simulink model "zlinearyzowany_dyskretny_model_dynamiczny"  (R2021a)
settings: Solver=VariableStepAuto  StartTime=0.0  StopTime=60  RelTol=1e-3
values from neighbouring files (symbols this model uses):
  a1 = 0.32    [Wartosci_w_zadaniu.m]    (also in zad_4.m)
  a2 = 0.45    [Wartosci_w_zadaniu.m]    (also in zad_4.m)
  a3 = -0.29    [Wartosci_w_zadaniu.m]    (also in zad_4.m)
  a4 = -0.1    [Wartosci_w_zadaniu.m]    (also in zad_4.m)
  K = 2    [Wartosci_w_zadaniu.m]    (also in zad_4.m)
  T = 1.5    [zad_4.m]
  T1 = 5    [Wartosci_w_zadaniu.m]    (also in zad_4.m)
  T2 = 8    [Wartosci_w_zadaniu.m]    (also in zad_4.m)
  u_0 = -0.85    [zad_5_i_6.m]
settings Model: Creator=ADMIN  LastModifiedBy=ADMIN

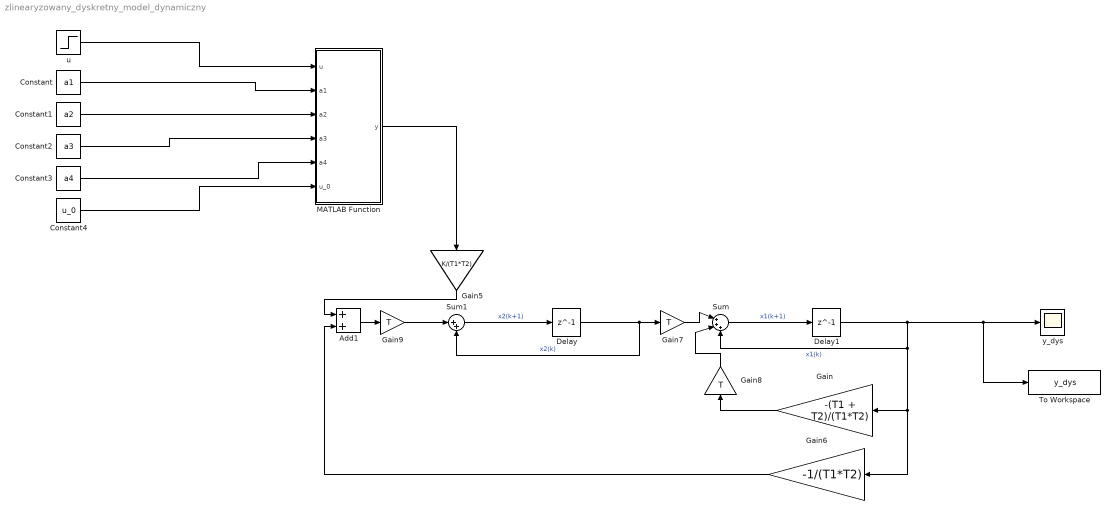
== system zlinearyzowany_dyskretny_model_dynamiczny ==
  Add1 : Sum
  Constant : Constant  Value=a1
  Constant1 : Constant  Value=a2
  Constant2 : Constant  Value=a3
  Constant3 : Constant  Value=a4
  Constant4 : Constant  Value=u_0
  Delay : Delay  DelayLength=1  InitialCondition=0  SampleTime=T
  Delay1 : Delay  DelayLength=1  InitialCondition=0  SampleTime=T
  Gain : Gain  Gain=-(T1 + T2)/(T1*T2)
  Gain5 : Gain  Gain=K/(T1*T2)
  Gain6 : Gain  Gain=-1/(T1*T2)
  Gain7 : Gain  Gain=T
  Gain8 : Gain  Gain=T
  Gain9 : Gain  Gain=T
  MATLAB Function : MATLAB Function  TreatAsAtomicUnit=on
  Sum : Sum  Inputs=|+++
  Sum1 : Sum  Inputs=|++
  To Workspace : ToWorkspace  VariableName=y_dys  SaveFormat=Structure With Time  SampleTime=T
  u : Step  SampleTime=0
  y_dys : Scope
  wires:
  Delay1/1 -> Sum/3, Gain6/1, Gain/1, To Workspace/1, y_dys/1  "x1(k)"
  Gain9/1 -> Sum1/1
  u/1 -> MATLAB Function/1(u)
  Gain8/1 -> Sum/2
  Sum1/1 -> Delay/1  "x2(k+1)"
  Gain/1 -> Gain8/1
  Gain5/1 -> Add1/1
  Add1/1 -> Gain9/1
  MATLAB Function/1(y) -> Gain5/1
  Gain6/1 -> Add1/2
  Gain7/1 -> Sum/1
  Delay/1 -> Sum1/2, Gain7/1  "x2(k)"
  Sum/1 -> Delay1/1  "x1(k+1)"
  Constant/1 -> MATLAB Function/2(a1)
  Constant4/1 -> MATLAB Function/6(u_0)
  Constant3/1 -> MATLAB Function/5(a4)
  Constant2/1 -> MATLAB Function/4(a3)
  Constant1/1 -> MATLAB Function/3(a2)

== matlab function zlinearyzowany_dyskretny_model_dynamiczny/MATLAB Function ==
  data: u input; y output; a1 input; a2 input; a3 input; a4 input; u_0 input
function y = fcn(u,a1,a2,a3,a4,u_0)
y = a1* u + a2*((u_0)^2 + 2*u_0*(u-u_0)) + a3*((u_0)^3 + 3*(u_0^2)*(u-u_0)) + a4*((u_0)^4 + 4*(u_0^3)*(u-u_0));
end
